simulink model "HaloMPCMatlab"  (R2019b)
settings: Solver=ode45  StartTime=0.0  StopTime=simTime  RelTol=1e-4
values from neighbouring files (symbols this model uses):
  a = zeros(2,1)    [initHaloSRMPC.m]
  b = zeros(2,1)    [initHaloSRMPC.m]
  c = zeros(2,1)    [Satellite.m]    (also in initHaloSRMPC.m)
  delta = 0.1    [initHaloSRMPC.m]
  disturbance = 0    [initHaloSRMPC.m]
  Gsc = 1360.8    [initHaloSRMPC.m]
  k = 0.1    [initHaloSRMPC.m]
  L2 = 1.1556    [Satellite.m]    (also in initHaloSRMPC.m)
  mu = 0.012149    [Satellite.m]    (also in initHaloSRMPC.m)
  Omega = 1.8636    [Satellite.m]    (also in initHaloSRMPC.m)
  Omega_z = Omega    (= 1.8636)    [Satellite.m]    (also in initHaloSRMPC.m)
  phi = 0    [initHaloSRMPC.m]
  satValue = inf    [initHaloSRMPC.m]
  sped = 300000    [initHaloSRMPC.m]
  srp = 0    [initHaloSRMPC.m]
  Ts = delta    (= 0.1)    [initHaloSRMPC.m]
  u0 = [0;0;0]    [initHaloSRMPC.m]
  x0 = [L2;0;0;0;0;0]    [initHaloSRMPC.m]
  zeta = 0.9252    [initHaloSRMPC.m]
libraries: mpclib x1
settings Model: Creator=mohd-  LastModifiedBy=mohd-

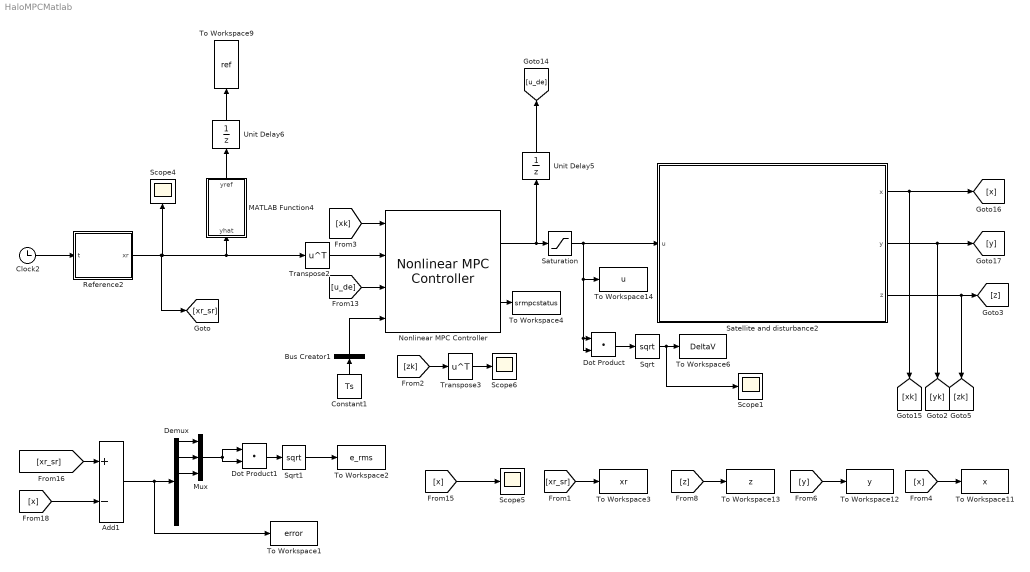
== system HaloMPCMatlab ==
  Add1 : Sum  Inputs=+-
  Bus Creator1 : BusCreator  Inputs=1  OutDataTypeStr=Bus: myBusObject  NonVirtualBus=on
      settings: InheritFromInputs=off
  Clock2 : Clock
  Constant1 : Constant  Value=Ts
  Demux : Demux  Outputs=6
  Dot Product : DotProduct  InputSameDT=on  OutDataTypeStr=Inherit: Inherit via internal rule
  Dot Product1 : DotProduct  InputSameDT=on  OutDataTypeStr=Inherit: Inherit via internal rule
  MATLAB Function4 : MATLAB Function  TreatAsAtomicUnit=on
  Mux : Mux  Inputs=3
  Nonlinear MPC Controller : mpclib/Nonlinear MPC Controller  SCDEnableBlockLinearizationSpecification=on  nlmpcobj=nlobjsr  UseObjectTs=off  TsControl=delta  md_enabled=off  mvtarget_enabled=off  param_enabled=on  cost_enabled=off  mvseq_enabled=off  stateseq_enabled=off  ovseq_enabled=off  slack_enabled=off  status_enabled=on  ov_min=off  ov_max=off  mv_min=off  mv_max=off  mvrate_min=off  mvrate_max=off  state_min=off  state_max=off  ov_weight=off  mv_weight=off  mvrate_weight=off  ecr_weight=off  nlp_initialize=off
      settings: SourceProductName=Model Predictive Control Toolbox
  Reference2 : MATLAB Function  TreatAsAtomicUnit=on
  Satellite and disturbance2 : Subsystem
  Saturation : Saturate  UpperLimit=satValue  LowerLimit=-satValue
  Scope{1,4..6} (4 alike) : Scope
  Sqrt : Sqrt  SaturateOnIntegerOverflow=on
  Sqrt1 : Sqrt  SaturateOnIntegerOverflow=on
  To Workspace1 : ToWorkspace  VariableName=error  SampleTime=10^-3
  To Workspace11 : ToWorkspace  VariableName=x  SampleTime=10^-3
  To Workspace12 : ToWorkspace  VariableName=y  SampleTime=10^-3
  To Workspace13 : ToWorkspace  VariableName=z  SampleTime=10^-3
  To Workspace14 : ToWorkspace  VariableName=u  SampleTime=10^-3
  To Workspace2 : ToWorkspace  VariableName=e_rms  SampleTime=10^-3
  To Workspace3 : ToWorkspace  VariableName=xr  SampleTime=10^-3
  To Workspace4 : ToWorkspace  VariableName=srmpcstatus  SampleTime=10^-3
  To Workspace6 : ToWorkspace  VariableName=DeltaV  SampleTime=10^-3
  To Workspace9 : ToWorkspace  VariableName=ref  SampleTime=delta
  Transpose2 : Math  Operator=transpose  SignedPower=off  SaturateOnIntegerOverflow=on
  Transpose3 : Math  Operator=transpose  SignedPower=off  SaturateOnIntegerOverflow=on
  Unit Delay5 : UnitDelay  InitialCondition=u0  SampleTime=delta  HasFrameUpgradeWarning=on
  Unit Delay6 : UnitDelay  InitialCondition=x0  SampleTime=delta  HasFrameUpgradeWarning=on
  wires:
  Nonlinear MPC Controller/1 -> Unit Delay5/1, Saturation/1
  Constant1/1 -> Bus Creator1/1
  [x] -> To Workspace11/1
  Satellite and disturbance2/2(y) -> [yk], [y]
  [z] -> To Workspace13/1
  Satellite and disturbance2/1("x ") -> [xk], [x]
  [x] -> Scope5/1
  Clock2/1 -> Reference2/1(t)
  [y] -> To Workspace12/1
  Unit Delay6/1 -> To Workspace9/1
  Unit Delay5/1 -> [u_de]
  [u_de] -> Nonlinear MPC Controller/3
  [zk] -> Transpose3/1
  Bus Creator1/1 -> Nonlinear MPC Controller/4
  Transpose3/1 -> Scope6/1
  Reference2/1(xr) -> [xr_sr], Scope4/1, MATLAB Function4/1(yhat), Transpose2/1
  Transpose2/1 -> Nonlinear MPC Controller/2
  MATLAB Function4/1(yref) -> Unit Delay6/1
  [xk] -> Nonlinear MPC Controller/1
  Sqrt1/1 -> To Workspace2/1
  Mux/1 -> Dot Product1/2, Dot Product1/1
  Demux/1 -> Mux/1
  Demux/3 -> Mux/3
  Add1/1 -> To Workspace1/1, Demux/1
  [x] -> Add1/2
  Demux/2 -> Mux/2
  [xr_sr] -> Add1/1
  Dot Product/1 -> Sqrt/1
  [xr_sr] -> To Workspace3/1
  Saturation/1 -> Satellite and disturbance2/1(u), Dot Product/1, Dot Product/2, To Workspace14/1
  Nonlinear MPC Controller/2 -> To Workspace4/1
  Sqrt/1 -> To Workspace6/1, Scope1/1
  Dot Product1/1 -> Sqrt1/1
  Satellite and disturbance2/3(z) -> [zk], [z]

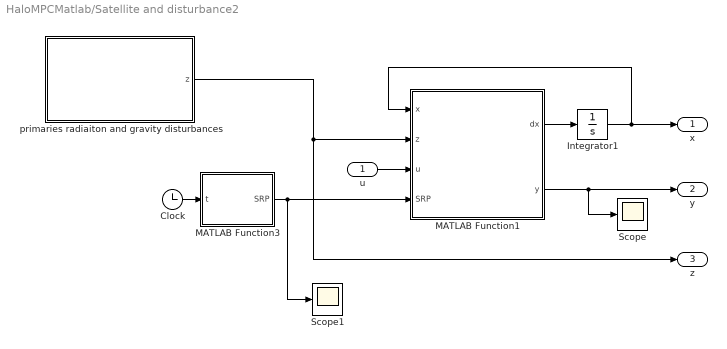
== system HaloMPCMatlab/Satellite and disturbance2 ==
  u : Inport
  Clock : Clock
  Integrator1 : Integrator  InitialCondition=x0
  MATLAB Function1 : MATLAB Function  TreatAsAtomicUnit=on
  MATLAB Function3 : MATLAB Function  TreatAsAtomicUnit=on
  Scope : Scope
  Scope1 : Scope
  primaries radiaiton and gravity disturbances : Subsystem
  "x " : Outport
  y : Outport  Port=2
  z : Outport  Port=3
  wires:
  Clock/1 -> MATLAB Function3/1(t)
  MATLAB Function1/1(dx) -> Integrator1/1
  MATLAB Function1/2(y) -> Scope/1, y/1
  u/1 -> MATLAB Function1/3(u)
  MATLAB Function3/1(SRP) -> Scope1/1, MATLAB Function1/4(SRP)
  Integrator1/1 -> "x "/1, MATLAB Function1/1(x)
  primaries radiaiton and gravity disturbances/1(z) -> z/1, MATLAB Function1/2(z)

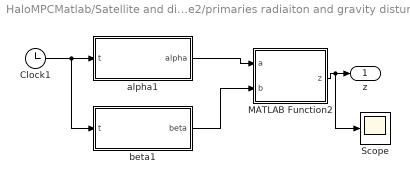
== system HaloMPCMatlab/Satellite and disturbance2/primaries radiaiton and gravity disturbances ==
  Clock1 : Clock
  MATLAB Function2 : MATLAB Function  TreatAsAtomicUnit=on
  Scope : Scope
  alpha1 : MATLAB Function  TreatAsAtomicUnit=on
  beta1 : MATLAB Function  TreatAsAtomicUnit=on
  z : Outport
  wires:
  Clock1/1 -> beta1/1(t), alpha1/1(t)
  beta1/1(beta) -> MATLAB Function2/2(b)
  alpha1/1(alpha) -> MATLAB Function2/1(a)
  MATLAB Function2/1(z) -> Scope/1, z/1

== matlab function HaloMPCMatlab/Satellite and disturbance2/MATLAB Function3 ==
  data: SRP output; srp parameter; Gsc parameter; sped parameter; zeta parameter; t input
function SRP = fcn(srp, Gsc, sped, zeta,t)

if srp == 1
    SRP = [(Gsc/sped)*(cos(zeta*t))^2;(Gsc/sped)*(sin(zeta*t))^2;0];
else
    SRP = [0;0;0];
end

== matlab function HaloMPCMatlab/MATLAB Function4 ==
  data: yhat input; yref output
function yref = fcn(yhat)

yref = yhat(:,1);

== matlab function HaloMPCMatlab/Reference2 ==
  data: t input; xr output; c parameter; Omega parameter; Omega_z parameter; L2 parameter; k parameter
function xr = refer(t,c,Omega,Omega_z,L2,k)
%#codegen

Seq = [L2;0;0;0;0;0];


ho1 = [(-k*(1-c(1)+Omega^2)/(2*Omega))*cos(Omega*t);
       k*sin(Omega*t);
       k*cos(Omega_z*t)];
   
diffho1 = [(k*(1-c(1)+Omega^2)/2)*sin(Omega*t);
           Omega*k*cos(Omega*t);
           -Omega_z*k*sin(Omega_z*t)];
      
xr = Seq + [ho1;diffho1];

== matlab function HaloMPCMatlab/Satellite and disturbance2/MATLAB Function1 ==
  data: x input; z input; dx output; u input; y output; mu parameter; SRP input
function [dx, y] = Satellite(x,z, u, mu, SRP)

x1 = x(1:3);
x2 = x(4:6);

M = [-1 0 0;
    0 -1 0;
    0 0 0];

N = [0 -1 0;
    1 0 0;
    0 0 0];

d1r = [-mu - z(4)/(1-mu);0;0];
d2r = [1-mu + z(4)/mu;0;0];

ed1 = x1 - d1r;
absed1 = sqrt(ed1(1)^2+ed1(2)^2+ed1(3)^2);
ed2 = x1 - d2r;
absed2 = sqrt(ed2(1)^2+ed2(2)^2+ed2(3)^2);

f1 = x2;
f2 = -M*x1 - 2*N*x2 - (2*M*x1 + 2*N*x2)*z(1) ...
           - M*x1*z(2) - N*x1*z(3) - ed1*(1 - mu)/absed1^3 ...
           - ed2*mu/absed2^3;
F = [f1; f2 + SRP];
G = [zeros(3); eye(3)];


dx = F + G*u;
y  = x1;

%% simplified model
% x_1 = x1(1);
% x_2 = x1(2);
% x_3 = x1(3);
% xd_1 = x2(1);
% xd_2 = x2(2);
% xd_3 = x2(3);
% % 
% f2 = [x_1 + 2*xd_2 - (mu*(mu + x_1 - 1))/((mu + x_1 - 1)^2 + x_2^2 + x_3^2)^(3/2) + ((mu + x_1)*(mu - 1))/((mu + x_1)^2 + x_2^2 + x_3^2)^(3/2);
%     x_2 - 2*xd_1 - (mu*x_2)/((mu + x_1 - 1)^2 + x_2^2 + x_3^2)^(3/2) + (x_2*(mu - 1))/((mu + x_1)^2 + x_2^2 + x_3^2)^(3/2);
%     (x_3*(mu - 1))/((mu + x_1)^2 + x_2^2 + x_3^2)^(3/2) - (mu*x_3)/((mu + x_1 - 1)^2 + x_2^2 + x_3^2)^(3/2)];
% 
% F = [x2; f2];
% 
% P44 = -2*((x_1+mu)^2+x_2^2+x_3^2)/((x_1+mu)^2+x_2^2+x_3^2)^(5/2) - 2*((x_1-1+mu)^2+x_2^2+x_3^2)/((x_1-1+mu)^2+x_2^2+x_3^2)^(5/2);
% P54 = 3*(x_2*(x_1+mu))/((x_1+mu)^2+x_2^2+x_3^2)^(5/2) - 3*(x_2*(x_1-1+mu))/((x_1-1+mu)^2+x_2^2+x_3^2)^(5/2);
% P64 = 3*(x_3*(x_1+mu))/((x_1+mu)^2+x_2^2+x_3^2)^(5/2) - 3*x_3*((x_1-1+mu))/((x_1-1+mu)^2+x_2^2+x_3^2)^(5/2);
% 
% P = [ 2*x_1 + 2*xd_2, x_1,  x_2, P44;
%     2*x_2 - 2*xd_1, x_2, -x_1, P54;
%     0,   0,    0, P64];
% 
% f = F + [zeros(3,4);P]*z;
% G = [zeros(3); eye(3)];
% dx = f + G*u;
% y = x1;

== matlab function HaloMPCMatlab/Satellite and disturbance2/primaries radiaiton and gravity disturbances/MATLAB Function2 ==
  data: a input; z output; b input; mu parameter; disturbance parameter
function z = z(a,b,mu, disturbance)
%#codegen
if disturbance == 1
    z = [b;mu*(1-mu)*a];
else
    z = zeros(4,1);
end

== matlab function HaloMPCMatlab/Satellite and disturbance2/primaries radiaiton and gravity disturbances/alpha1 ==
  data: t input; alpha output; a parameter; phi parameter; e parameter
function alpha = a(t,a,phi,e)
%#codegen

a1 = a(1)*e*cos(t+phi);
alpha = a1;

== matlab function HaloMPCMatlab/Satellite and disturbance2/primaries radiaiton and gravity disturbances/beta1 ==
  data: t input; beta output; b parameter; phi parameter; e parameter
function beta = b(t,b,phi,e)
%#codegen
b1 = b(1)*e*cos(t+phi);
bd = -b(1)*e*sin(t+phi);
beta = [b1;0;bd];
